simulink model "kociolsimulinkskok"  (R2024a)
settings: Solver=ode45  StartTime=0.0  StopTime=3000  MaxStep=1  RelTol=1e-3  AbsTol=1e-6
values from neighbouring files (symbols this model uses):
  cpw = 4190    [aparam1.m]
  Cvg = (no*Vg)*row*cpw/skala    (= 3421.83333333)    [aparam1.m]
  Cvk = (Vk)*row*cpw/skala    (= 3421.83333333)    [aparam1.m]
  Cvws = (Cvw +Cvs) / 2    [aparam1.m]
  czas_skok = 500    [2punktowazn.m]    (also in KociolPom1CvwCvgCvs_skrypt.m; KociolPom1CvwCvg_skrypt.m; kociolsimulinkskokjednostkowy.m; stycznazn.m)
  dFg = 0*FgN    [2punktowazn.m]    (also in KociolPom1CvwCvgCvs_skrypt.m; KociolPom1CvwCvg_skrypt.m; kociolsimulinkskokjednostkowy.m = 0; stycznazn.m)
  dQk = 0.1 * QkN    (= 200)    [2punktowazn.m]    (also in KociolPom1CvwCvgCvs_skrypt.m; KociolPom1CvwCvg_skrypt.m = 400; kociolsimulinkskokjednostkowy.m; stycznazn.m = 0)
  dQt = 0    [2punktowazn.m]    (also in KociolPom1CvwCvgCvs_skrypt.m; KociolPom1CvwCvg_skrypt.m; kociolsimulinkskokjednostkowy.m; stycznazn.m = 200)
  dTzew = 0    [2punktowazn.m]    (also in KociolPom1CvwCvgCvs_skrypt.m; KociolPom1CvwCvg_skrypt.m; kociolsimulinkskokjednostkowy.m; stycznazn.m)
  Fg0 = FgN    [2punktowazn.m]    (also in KociolPom1CvwCvgCvs_skrypt.m; KociolPom1CvwCvg_skrypt.m; kociolsimulinkskokjednostkowy.m; stycznazn.m)
  final_value = +2    (= 2)    [2punktowazn.m]    (also in stycznazn.m = 0)
  K = (y_koncowe - y_poczatkowe) / wejscie_skok    [2punktowazn.m]    (also in stycznazn.m = 1)
  Kcg = QgN/(TgpN-TwewN)    (= 40)    [2punktowazn.m]    (also in KociolPom1CvwCvgCvs_skrypt.m; KociolPom1CvwCvg_skrypt.m; kociolsimulinkskokjednostkowy.m; stycznazn.m)
  Kcw = QgN/(TwewN-TzewN)    (= 50)    [2punktowazn.m]    (also in KociolPom1CvwCvgCvs_skrypt.m = 133.333333333; KociolPom1CvwCvg_skrypt.m; kociolsimulinkskokjednostkowy.m; stycznazn.m)
  Ki_ZN = Kp_ZN / Ti_ZN    [2punktowazn.m]    (also in stycznazn.m = Ki_SIMC)
  Kp_ZN = 0.9 * T / (K * T0)    [2punktowazn.m]    (also in stycznazn.m = Kp_SIMC)
  Qk0 = QkN    (= 2000)    [2punktowazn.m]    (also in KociolPom1CvwCvgCvs_skrypt.m; KociolPom1CvwCvg_skrypt.m = 0; kociolsimulinkskokjednostkowy.m; stycznazn.m)
  Qt0 = 0    [2punktowazn.m]    (also in KociolPom1CvwCvgCvs_skrypt.m; KociolPom1CvwCvg_skrypt.m; kociolsimulinkskokjednostkowy.m; stycznazn.m)
  T = 1.5 * (t_63_2 - t_28_3)    [2punktowazn.m]    (also in stycznazn.m = T_styczna)
  T0 = 2.33 * t_28_3 - 1.33 * t_63_2    [2punktowazn.m]    (also in stycznazn.m = T0_styczna)
  Tgp0 = x0(2)    [2punktowazn.m]    (also in KociolPom1CvwCvgCvs_skrypt.m; KociolPom1CvwCvg_skrypt.m; kociolsimulinkskokjednostkowy.m = 70; stycznazn.m = 70)
  Tkz0 = x0(3)    [2punktowazn.m]    (also in KociolPom1CvwCvgCvs_skrypt.m = x0(4); KociolPom1CvwCvg_skrypt.m; kociolsimulinkskokjednostkowy.m = Qk0/(cpw*Fk0) + Tgp0; stycznazn.m = Qk0/(cpw*Fk0) + Tgp0)
  To = 20*60/skala    (= 20)    [aparam1.m]
  Twew0 = x0(1)    [2punktowazn.m]    (also in KociolPom1CvwCvgCvs_skrypt.m; KociolPom1CvwCvg_skrypt.m; kociolsimulinkskokjednostkowy.m = 20; stycznazn.m = 20)
  Tzew0 = TzewN+0    (= -20)    [2punktowazn.m]    (also in KociolPom1CvwCvgCvs_skrypt.m; KociolPom1CvwCvg_skrypt.m; kociolsimulinkskokjednostkowy.m; stycznazn.m)
libraries: slpidlib x2
settings Model: Creator=ac  LastModifiedBy=mateu
settings SolverCC: AutoScaleAbsTol=off  AlgebraicLoopSolver=TrustRegion
settings DataIOCC: SaveFormat=Array  SignalLoggingSaveFormat=ModelDataLogs  ReturnWorkspaceOutputs=off
settings OptimizationCC: BlockReduction=off  BooleanDataType=off  ExpressionDepthLimit=2147483647  LifeSpan=inf
settings DebuggingCC: SaveWithParameterizedLinksMsg=none  UnderspecifiedInitializationDetection=Classic  MergeDetectMultiDrivingBlocksExec=none  SignalResolutionControl=TryResolveAllWithWarning  MultiTaskDSMMsg=warning  MultiTaskCondExecSysMsg=none  FcnCallInpInsideContextMsg=warning  UnconnectedInputMsg=warning  UnconnectedOutputMsg=warning  UnconnectedLineMsg=warning  StateNameClashWarn=warning  SFUnexpectedBacktrackingDiag=warning  SFNoUnconditionalDefaultTransitionDiag=warning  SFExecutionAtInitializationDiag=none  ArithmeticOperatorsInVariantConditions=warning
settings HardwareCC: ProdBitPerPointer=32  ProdBitPerSizeT=32  ProdBitPerPtrDiffT=32  ProdLargestAtomicFloat=None  ProdIntDivRoundTo=Undefined  ProdEndianess=Unspecified  ProdWordSize=32  ProdHWDeviceType=32-bit Generic  TargetUnknown=on
settings ModelReferenceCC: PropagateSignalLabelsOutOfModel=off
settings SFSimCC: SimUseLocalCustomCode=off  CustomCodeUndefinedFunction=UseInterfaceOnly
settings RTWCC: RTWUseLocalCustomCode=off  GPUComputeCapability=3.5
settings CodeAppCC: StateflowObjectComments=on
settings GRTTargetCC: TargetLangStandard=C89/C90 (ANSI)  CombineOutputUpdateFcns=off  GRTInterface=on
settings ConfigComp: CovMetricSettings=dw  CovSaveCumulativeToWorkspaceVar=on  CovSaveSingleToWorkspaceVar=on  CovExternalEMLEnable=off

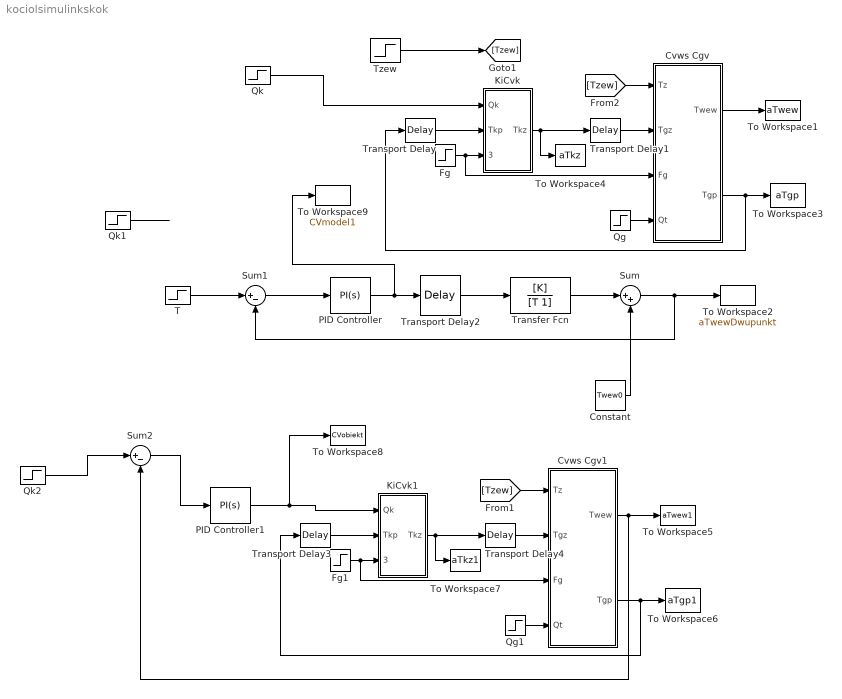
== system kociolsimulinkskok ==
  Constant : Constant  Value=Twew0
  Cvws Cgv : Subsystem
  Cvws Cgv1 : Subsystem
  Fg : Step  Time=czas_skok  Before=Fg0  After=Fg0+dFg  SampleTime=0
  Fg1 : Step  Time=czas_skok  Before=Fg0  After=Fg0+dFg  SampleTime=0
  KiCvk : Subsystem  mask{cpw=cpw, Cvk=Cvk, Tkz0=Tkz0}
  KiCvk1 : Subsystem  mask{cpw=cpw, Cvk=Cvk, Tkz0=Tkz0}
  PID Controller : slpidlib/PID Controller  Controller=PI  Form=Parallel  TimeDomain=Continuous-time  UseExternalTs=off  SampleTime=-1  IntegratorMethod=Forward Euler  FilterMethod=Forward Euler  ControllerParametersSource=internal  P=Kp_ZN  I=Ki_ZN  UseKiTs=off  D=0  UseExternalDerivativeSource=off  N=100  UseFilter=on  TunerSelectOption=Transfer Function Based (PID Tuner App)  InitialConditionSource=internal  InitialConditionForIntegrator=0  InitialConditionForFilter=0  DifferentiatorICPrevScaledInput=0  ExternalReset=none  TrackingMode=off  Kt=1  LimitOutput=off  SatLimitsSource=internal  UpperSaturationLimit=inf  LowerSaturationLimit=-inf  LinearizeAsGain=on  AntiWindupMode=none  Kb=1  LimitIntegrator=off  UpperIntegratorSaturationLimit=inf  LowerIntegratorSaturationLimit=-inf  POutMin=[]  POutMax=[]  IOutMin=[]  IOutMax=[]  DOutMin=[]  DOutMax=[]  NOutMin=[]  NOutMax=[]  SumOutMin=[]  SumOutMax=[]  SaturationOutMin=[]  SaturationOutMax=[]  PParamMin=[]  PParamMax=[]  IParamMin=[]  IParamMax=[]  DParamMin=[]  DParamMax=[]  NParamMin=[]  NParamMax=[]  KbParamMin=[]  KbParamMax=[]  KtParamMin=[]  KtParamMax=[]  KbOutMin=[]  KbOutMax=[]  KtOutMin=[]  KtOutMax=[]  IntegratorOutMin=[]  IntegratorOutMax=[]  FilterOutMin=[]  FilterOutMax=[]  SumI1OutMin=[]  SumI1OutMax=[]  SumI2OutMin=[]  SumI2OutMax=[]  SumI3OutMin=[]  SumI3OutMax=[]  SumI4OutMin=[]  SumI4OutMax=[]  SumDOutMin=[]  SumDOutMax=[]  DifferentiatorOutMin=[]  DifferentiatorOutMax=[]  FilterDiffOutCoefMin=[]  FilterDiffOutCoefMax=[]  ReciprocalOutMin=[]  ReciprocalOutMax=[]  SumDenOutMin=[]  SumDenOutMax=[]  SumNumOutMin=[]  SumNumOutMax=[]  DivideOutMin=[]  DivideOutMax=[]  UdiffTsProdOutMin=[]  UdiffTsProdOutMax=[]  NTsProdOutMin=[]  NTsProdOutMax=[]  UintegralTsProdOutMin=[]  UintegralTsProdOutMax=[]  UngainTsProdOutMin=[]  UngainTsProdOutMax=[]  ClampingZeroOutDataTypeStr=Inherit: Inherit via back propagation  ClampingZeroOutMin=[]  ClampingZeroOutMax=[]  FilterDenConstantOutDataTypeStr=Inherit: Inherit via back propagation  FilterDenConstantOutMin=[]  FilterDenConstantOutMax=[]  PCopyOutDataTypeStr=Inherit: Inherit via back propagation  PCopyOutMin=[]  PCopyOutMax=[]  NCopyOutDataTypeStr=Inherit: Inherit via back propagation  NCopyOutMin=[]  NCopyOutMax=[]  IntegratorContinuousStateAttributes=''  IntegratorStateMustResolveToSignalObject=off  IntegratorRTWStateStorageClass=Auto  FilterContinuousStateAttributes=''  FilterStateMustResolveToSignalObject=off  FilterRTWStateStorageClass=Auto  ParallelPVariant=InternalParameters  IdealPVariant=Disabled  IVariant=InternalParameters  DVariant=Disabled  IntegratorVariant=Continuous  SatVariant=Disabled  AWVariant=Passthrough  PCopyVariant=Disabled  TRVariant=Disabled  FdbkBlocksVariant=Forward  IdealPFdbkVariant=Disabled  SatFdbkVariant=Disabled  DerivativeFilterVariant=Disabled  NVariant=Disabled  NCopyVariant=Disabled_SignalSpec  FilterICVariant=Disabled  IntegratorICVariant=InternalICs  ExternalResetVariant=Disabled  TRSumVariant=Passthrough  SumFdbkVariant=Disabled  SumVariant=Sum_PI  TsampFilterVariant=InternalTs  TsampNgainVariant=Passthrough  TsampIntegralVariant=Disabled_SignalSpec  ExternalSaturationOutDataTypeStr=Inherit: Same as second input  DerivativeSourceVariant=Disabled
  PID Controller1 : slpidlib/PID Controller  Controller=PI  Form=Parallel  TimeDomain=Continuous-time  UseExternalTs=off  SampleTime=-1  IntegratorMethod=Forward Euler  FilterMethod=Forward Euler  ControllerParametersSource=internal  P=Kp_ZN  I=Ki_ZN  UseKiTs=off  D=0  UseExternalDerivativeSource=off  N=100  UseFilter=on  TunerSelectOption=Transfer Function Based (PID Tuner App)  InitialConditionSource=internal  InitialConditionForIntegrator=Qk0  InitialConditionForFilter=0  DifferentiatorICPrevScaledInput=0  ExternalReset=none  TrackingMode=off  Kt=1  LimitOutput=off  SatLimitsSource=internal  UpperSaturationLimit=inf  LowerSaturationLimit=-inf  LinearizeAsGain=on  AntiWindupMode=none  Kb=1  LimitIntegrator=off  UpperIntegratorSaturationLimit=inf  LowerIntegratorSaturationLimit=-inf  POutMin=[]  POutMax=[]  IOutMin=[]  IOutMax=[]  DOutMin=[]  DOutMax=[]  NOutMin=[]  NOutMax=[]  SumOutMin=[]  SumOutMax=[]  SaturationOutMin=[]  SaturationOutMax=[]  PParamMin=[]  PParamMax=[]  IParamMin=[]  IParamMax=[]  DParamMin=[]  DParamMax=[]  NParamMin=[]  NParamMax=[]  KbParamMin=[]  KbParamMax=[]  KtParamMin=[]  KtParamMax=[]  KbOutMin=[]  KbOutMax=[]  KtOutMin=[]  KtOutMax=[]  IntegratorOutMin=[]  IntegratorOutMax=[]  FilterOutMin=[]  FilterOutMax=[]  SumI1OutMin=[]  SumI1OutMax=[]  SumI2OutMin=[]  SumI2OutMax=[]  SumI3OutMin=[]  SumI3OutMax=[]  SumI4OutMin=[]  SumI4OutMax=[]  SumDOutMin=[]  SumDOutMax=[]  DifferentiatorOutMin=[]  DifferentiatorOutMax=[]  FilterDiffOutCoefMin=[]  FilterDiffOutCoefMax=[]  ReciprocalOutMin=[]  ReciprocalOutMax=[]  SumDenOutMin=[]  SumDenOutMax=[]  SumNumOutMin=[]  SumNumOutMax=[]  DivideOutMin=[]  DivideOutMax=[]  UdiffTsProdOutMin=[]  UdiffTsProdOutMax=[]  NTsProdOutMin=[]  NTsProdOutMax=[]  UintegralTsProdOutMin=[]  UintegralTsProdOutMax=[]  UngainTsProdOutMin=[]  UngainTsProdOutMax=[]  ClampingZeroOutDataTypeStr=Inherit: Inherit via back propagation  ClampingZeroOutMin=[]  ClampingZeroOutMax=[]  FilterDenConstantOutDataTypeStr=Inherit: Inherit via back propagation  FilterDenConstantOutMin=[]  FilterDenConstantOutMax=[]  PCopyOutDataTypeStr=Inherit: Inherit via back propagation  PCopyOutMin=[]  PCopyOutMax=[]  NCopyOutDataTypeStr=Inherit: Inherit via back propagation  NCopyOutMin=[]  NCopyOutMax=[]  IntegratorContinuousStateAttributes=''  IntegratorStateMustResolveToSignalObject=off  IntegratorRTWStateStorageClass=Auto  FilterContinuousStateAttributes=''  FilterStateMustResolveToSignalObject=off  FilterRTWStateStorageClass=Auto  ParallelPVariant=InternalParameters  IdealPVariant=Disabled  IVariant=InternalParameters  DVariant=Disabled  IntegratorVariant=Continuous  SatVariant=Disabled  AWVariant=Passthrough  PCopyVariant=Disabled  TRVariant=Disabled  FdbkBlocksVariant=Forward  IdealPFdbkVariant=Disabled  SatFdbkVariant=Disabled  DerivativeFilterVariant=Disabled  NVariant=Disabled  NCopyVariant=Disabled_SignalSpec  FilterICVariant=Disabled  IntegratorICVariant=InternalICs  ExternalResetVariant=Disabled  TRSumVariant=Passthrough  SumFdbkVariant=Disabled  SumVariant=Sum_PI  TsampFilterVariant=InternalTs  TsampNgainVariant=Passthrough  TsampIntegralVariant=Disabled_SignalSpec  ExternalSaturationOutDataTypeStr=Inherit: Same as second input  DerivativeSourceVariant=Disabled
  Qg : Step  Time=czas_skok  Before=Qt0  After=Qt0+dQt  SampleTime=0
  Qg1 : Step  Time=czas_skok  Before=Qt0  After=Qt0+dQt  SampleTime=0
  Qk : Step  Time=czas_skok  Before=Qk0  After=Qk0+dQk  SampleTime=0
  Qk1 : Step  Time=czas_skok  After=dQk  SampleTime=0
  Qk2 : Step  Time=czas_skok  Before=Twew0  After=Twew0+final_value  SampleTime=0
  Sum : Sum  Inputs=|++
  Sum1 : Sum  Inputs=|+-
  Sum2 : Sum  Inputs=|+-
  T : Step  Time=czas_skok  Before=Twew0  After=Twew0+final_value  SampleTime=0
  To Workspace1 : ToWorkspace  VariableName=aTwew  SampleTime=-1
  To Workspace2 : ToWorkspace  VariableName=aTwewDwupunkt  SampleTime=-1
  To Workspace3 : ToWorkspace  VariableName=aTgp  SampleTime=-1
  To Workspace4 : ToWorkspace  VariableName=aTkz  SampleTime=-1
  To Workspace5 : ToWorkspace  VariableName=aTwew1  SampleTime=-1
  To Workspace6 : ToWorkspace  VariableName=aTgp1  SampleTime=-1
  To Workspace7 : ToWorkspace  VariableName=aTkz1  SampleTime=-1
  To Workspace8 : ToWorkspace  VariableName=CVobiekt  SampleTime=-1
  To Workspace9 : ToWorkspace  VariableName=CVmodel1  SampleTime=-1
  Transfer Fcn : TransferFcn  Numerator=[K]  Denominator=[T 1]
  Transport Delay : TransportDelay  DelayTime=To  InitialOutput=Tgp0
  Transport Delay1 : TransportDelay  DelayTime=To  InitialOutput=Tkz0
  Transport Delay2 : TransportDelay  DelayTime=T0
  Transport Delay3 : TransportDelay  DelayTime=To  InitialOutput=Tgp0
  Transport Delay4 : TransportDelay  DelayTime=To  InitialOutput=Tkz0
  Tzew : Step  Time=czas_skok  Before=Tzew0  After=Tzew0+dTzew  SampleTime=0
  wires:
  Fg/1 -> KiCvk/3(Fgm), Cvws Cgv/3(Fg)
  Transport Delay/1 -> KiCvk/2(Tkp)
  Qg/1 -> Cvws Cgv/4(Qt)
  Cvws Cgv/1(Twew) -> To Workspace1/1
  Cvws Cgv/2(Tgp) -> To Workspace3/1, Transport Delay/1
  Transport Delay1/1 -> Cvws Cgv/2(Tgz)
  [Tzew] -> Cvws Cgv/1(Tz)
  KiCvk/1(Tkz) -> Transport Delay1/1, To Workspace4/1
  Qk/1 -> KiCvk/1(Qk)
  Tzew/1 -> [Tzew]
  Transfer Fcn/1 -> Sum/1
  Transport Delay2/1 -> Transfer Fcn/1
  Qk1/1 -> ?
  Constant/1 -> Sum/2
  Sum/1 -> Sum1/2, To Workspace2/1
  Sum1/1 -> PID Controller/1
  T/1 -> Sum1/1
  PID Controller/1 -> To Workspace9/1, Transport Delay2/1
  Fg1/1 -> KiCvk1/3(Fgm), Cvws Cgv1/3(Fg)
  Transport Delay4/1 -> Cvws Cgv1/2(Tgz)
  KiCvk1/1(Tkz) -> Transport Delay4/1, To Workspace7/1
  ? -> ?
  [Tzew] -> Cvws Cgv1/1(Tz)
  Qg1/1 -> Cvws Cgv1/4(Qt)
  Transport Delay3/1 -> KiCvk1/2(Tkp)
  Cvws Cgv1/1(Twew) -> To Workspace5/1, Sum2/2
  Cvws Cgv1/2(Tgp) -> To Workspace6/1, Transport Delay3/1
  Qk2/1 -> Sum2/1
  PID Controller1/1 -> To Workspace8/1, KiCvk1/1(Qk)
  Sum2/1 -> PID Controller1/1

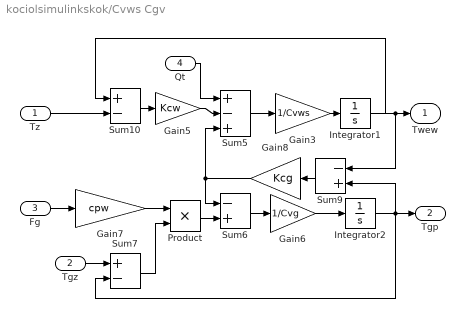
== system kociolsimulinkskok/Cvws Cgv ==
  Tz : Inport
  Tgz : Inport  Port=2
  Fg : Inport  Port=3
  Qt : Inport  Port=4
  Gain3 : Gain  Gain=1/Cvws  SaturateOnIntegerOverflow=on  OutDataTypeStr=Inherit: Same as input  ParamDataTypeStr=Inherit: Same as input
  Gain5 : Gain  Gain=Kcw  SaturateOnIntegerOverflow=on  OutDataTypeStr=Inherit: Same as input  ParamDataTypeStr=Inherit: Same as input
  Gain6 : Gain  Gain=1/Cvg  SaturateOnIntegerOverflow=on  OutDataTypeStr=Inherit: Same as input  ParamDataTypeStr=Inherit: Same as input
  Gain7 : Gain  Gain=cpw  SaturateOnIntegerOverflow=on  OutDataTypeStr=Inherit: Same as input  ParamDataTypeStr=Inherit: Same as input
  Gain8 : Gain  Gain=Kcg  SaturateOnIntegerOverflow=on  OutDataTypeStr=Inherit: Same as input  ParamDataTypeStr=Inherit: Same as input
  Integrator1 : Integrator  InitialCondition=Twew0
  Integrator2 : Integrator  InitialCondition=Tgp0
  Product : Product  InputSameDT=on  RndMeth=Zero  SaturateOnIntegerOverflow=on  OutDataTypeStr=Inherit: Same as first input
  Sum10 : Sum  Inputs=+-  InputSameDT=on  SaturateOnIntegerOverflow=on  OutDataTypeStr=Inherit: Same as first input
  Sum5 : Sum  Inputs=+-+  InputSameDT=on  SaturateOnIntegerOverflow=on  OutDataTypeStr=Inherit: Same as first input
  Sum6 : Sum  Inputs=-+  InputSameDT=on  SaturateOnIntegerOverflow=on  OutDataTypeStr=Inherit: Same as first input
  Sum7 : Sum  Inputs=+-  InputSameDT=on  SaturateOnIntegerOverflow=on  OutDataTypeStr=Inherit: Same as first input
  Sum9 : Sum  Inputs=-+  InputSameDT=on  SaturateOnIntegerOverflow=on  OutDataTypeStr=Inherit: Same as first input
  Twew : Outport
  Tgp : Outport  Port=2
  wires:
  Sum5/1 -> Gain3/1
  Sum6/1 -> Gain6/1
  Gain7/1 -> Product/1
  Sum7/1 -> Product/2
  Product/1 -> Sum6/2
  Gain6/1 -> Integrator2/1
  Integrator2/1 -> Sum7/2, Sum9/2, Tgp/1
  Sum9/1 -> Gain8/1
  Gain3/1 -> Integrator1/1
  Integrator1/1 -> Sum9/1, Sum10/1, Twew/1
  Sum10/1 -> Gain5/1
  Gain8/1 -> Sum6/1, Sum5/3
  Gain5/1 -> Sum5/2
  Qt/1 -> Sum5/1
  Fg/1 -> Gain7/1
  Tgz/1 -> Sum7/1
  Tz/1 -> Sum10/2

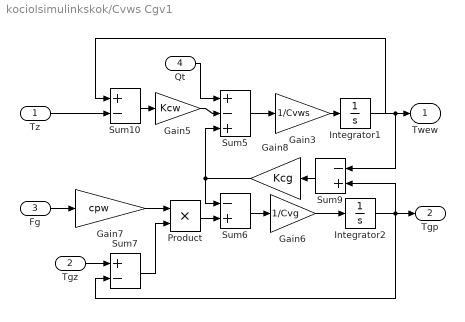
== system kociolsimulinkskok/Cvws Cgv1 ==
  Tz : Inport
  Tgz : Inport  Port=2
  Fg : Inport  Port=3
  Qt : Inport  Port=4
  Gain3 : Gain  Gain=1/Cvws  SaturateOnIntegerOverflow=on  OutDataTypeStr=Inherit: Same as input  ParamDataTypeStr=Inherit: Same as input
  Gain5 : Gain  Gain=Kcw  SaturateOnIntegerOverflow=on  OutDataTypeStr=Inherit: Same as input  ParamDataTypeStr=Inherit: Same as input
  Gain6 : Gain  Gain=1/Cvg  SaturateOnIntegerOverflow=on  OutDataTypeStr=Inherit: Same as input  ParamDataTypeStr=Inherit: Same as input
  Gain7 : Gain  Gain=cpw  SaturateOnIntegerOverflow=on  OutDataTypeStr=Inherit: Same as input  ParamDataTypeStr=Inherit: Same as input
  Gain8 : Gain  Gain=Kcg  SaturateOnIntegerOverflow=on  OutDataTypeStr=Inherit: Same as input  ParamDataTypeStr=Inherit: Same as input
  Integrator1 : Integrator  InitialCondition=Twew0
  Integrator2 : Integrator  InitialCondition=Tgp0
  Product : Product  InputSameDT=on  RndMeth=Zero  SaturateOnIntegerOverflow=on  OutDataTypeStr=Inherit: Same as first input
  Sum10 : Sum  Inputs=+-  InputSameDT=on  SaturateOnIntegerOverflow=on  OutDataTypeStr=Inherit: Same as first input
  Sum5 : Sum  Inputs=+-+  InputSameDT=on  SaturateOnIntegerOverflow=on  OutDataTypeStr=Inherit: Same as first input
  Sum6 : Sum  Inputs=-+  InputSameDT=on  SaturateOnIntegerOverflow=on  OutDataTypeStr=Inherit: Same as first input
  Sum7 : Sum  Inputs=+-  InputSameDT=on  SaturateOnIntegerOverflow=on  OutDataTypeStr=Inherit: Same as first input
  Sum9 : Sum  Inputs=-+  InputSameDT=on  SaturateOnIntegerOverflow=on  OutDataTypeStr=Inherit: Same as first input
  Twew : Outport
  Tgp : Outport  Port=2
  wires:
  Sum5/1 -> Gain3/1
  Sum6/1 -> Gain6/1
  Gain7/1 -> Product/1
  Sum7/1 -> Product/2
  Product/1 -> Sum6/2
  Gain6/1 -> Integrator2/1
  Integrator2/1 -> Sum7/2, Sum9/2, Tgp/1
  Sum9/1 -> Gain8/1
  Gain3/1 -> Integrator1/1
  Integrator1/1 -> Sum9/1, Sum10/1, Twew/1
  Sum10/1 -> Gain5/1
  Gain8/1 -> Sum6/1, Sum5/3
  Gain5/1 -> Sum5/2
  Qt/1 -> Sum5/1
  Fg/1 -> Gain7/1
  Tgz/1 -> Sum7/1
  Tz/1 -> Sum10/2

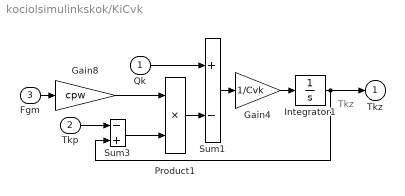
== system kociolsimulinkskok/KiCvk ==
  note: Tkz
  Qk : Inport
  Tkp : Inport  Port=2
  Fgm : Inport  Port=3
  Gain4 : Gain  Gain=1/Cvk  SaturateOnIntegerOverflow=on  OutDataTypeStr=Inherit: Same as input  ParamDataTypeStr=Inherit: Same as input
  Gain8 : Gain  Gain=cpw  SaturateOnIntegerOverflow=on  OutDataTypeStr=Inherit: Same as input  ParamDataTypeStr=Inherit: Same as input
  Integrator1 : Integrator  InitialCondition=Tkz0
  Product1 : Product  Inputs=**  InputSameDT=on  RndMeth=Zero  SaturateOnIntegerOverflow=on  OutDataTypeStr=Inherit: Same as first input
  Sum1 : Sum  Inputs=+-  InputSameDT=on  SaturateOnIntegerOverflow=on  OutDataTypeStr=Inherit: Same as first input
  Sum3 : Sum  Inputs=-+  InputSameDT=on  SaturateOnIntegerOverflow=on  OutDataTypeStr=Inherit: Same as first input
  Tkz : Outport
  wires:
  Tkp/1 -> Sum3/1
  Integrator1/1 -> Sum3/2, Tkz/1
  Product1/1 -> Sum1/2
  Sum1/1 -> Gain4/1
  Gain4/1 -> Integrator1/1
  Qk/1 -> Sum1/1
  Gain8/1 -> Product1/1
  Sum3/1 -> Product1/2
  Fgm/1 -> Gain8/1

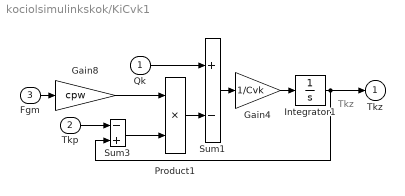
== system kociolsimulinkskok/KiCvk1 ==
  note: Tkz
  Qk : Inport
  Tkp : Inport  Port=2
  Fgm : Inport  Port=3
  Gain4 : Gain  Gain=1/Cvk  SaturateOnIntegerOverflow=on  OutDataTypeStr=Inherit: Same as input  ParamDataTypeStr=Inherit: Same as input
  Gain8 : Gain  Gain=cpw  SaturateOnIntegerOverflow=on  OutDataTypeStr=Inherit: Same as input  ParamDataTypeStr=Inherit: Same as input
  Integrator1 : Integrator  InitialCondition=Tkz0
  Product1 : Product  Inputs=**  InputSameDT=on  RndMeth=Zero  SaturateOnIntegerOverflow=on  OutDataTypeStr=Inherit: Same as first input
  Sum1 : Sum  Inputs=+-  InputSameDT=on  SaturateOnIntegerOverflow=on  OutDataTypeStr=Inherit: Same as first input
  Sum3 : Sum  Inputs=-+  InputSameDT=on  SaturateOnIntegerOverflow=on  OutDataTypeStr=Inherit: Same as first input
  Tkz : Outport
  wires:
  Tkp/1 -> Sum3/1
  Integrator1/1 -> Sum3/2, Tkz/1
  Product1/1 -> Sum1/2
  Sum1/1 -> Gain4/1
  Gain4/1 -> Integrator1/1
  Qk/1 -> Sum1/1
  Gain8/1 -> Product1/1
  Sum3/1 -> Product1/2
  Fgm/1 -> Gain8/1
